simulink model "sdf_pi_test"  (R2018b)
settings: Solver=FixedStepAuto  StartTime=0.0  StopTime=60  FixedStep=tSample  RelTol=1e-3
PreLoadFcn:
  | init
values from neighbouring files (symbols this model uses):
  tSample = 1/fSample    (= 0.1)    [Ekf.m]    (also in init.m)
undefined symbols (not defined in the file or in its folder): X, Y, Z
libraries: robotlib x2
settings Model: Creator=HannesDittmann  LastModifiedBy=HannesDittmann

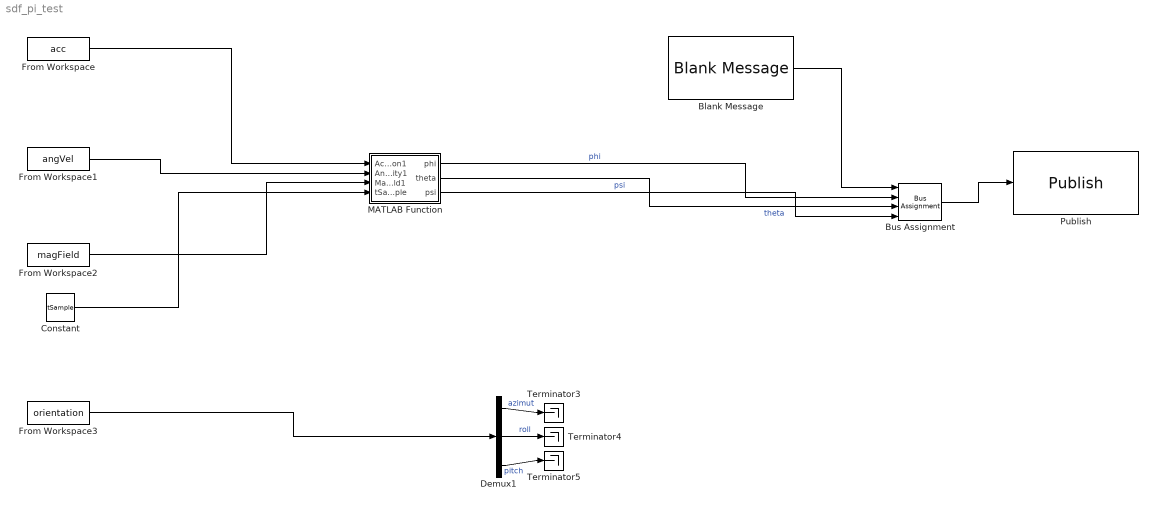
== system sdf_pi_test ==
  Blank Message : robotlib/Blank Message  messageClass=Message  entityType=geometry_msgs/Point  messageType=geometry_msgs/Point  SampleTime=inf
      settings: SourceProductBaseCode=RO
  Bus Assignment : BusAssignment  AssignedSignals=X,Y,Z
  Constant : Constant  Value=tSample
  Demux1 : Demux  Outputs=3
  From Workspace : FromWorkspace  VariableName=acc  Interpolate=off  OutputAfterFinalValue=Setting to zero
  From Workspace1 : FromWorkspace  VariableName=angVel  Interpolate=off  OutputAfterFinalValue=Setting to zero
  From Workspace2 : FromWorkspace  VariableName=magField  Interpolate=off  OutputAfterFinalValue=Setting to zero
  From Workspace3 : FromWorkspace  VariableName=orientation  Interpolate=off  OutputAfterFinalValue=Setting to zero
  MATLAB Function : MATLAB Function  TreatAsAtomicUnit=on
  Publish : robotlib/Publish  topicSource=Specify your own  topic=/euler  messageType=geometry_msgs/Point  messageQueueLength=1
      settings: SourceProductBaseCode=RO
  Terminator3 : Terminator
  Terminator4 : Terminator
  Terminator5 : Terminator
  wires:
  From Workspace/1 -> MATLAB Function/1(Acceleration1)
  From Workspace1/1 -> MATLAB Function/2(AngularVelocity1)
  From Workspace2/1 -> MATLAB Function/3(MagneticField1)
  Constant/1 -> MATLAB Function/4(tSample)
  From Workspace3/1 -> Demux1/1
  MATLAB Function/1(phi) -> Bus Assignment/2  "phi"
  MATLAB Function/2(theta) -> Bus Assignment/3  "theta"
  MATLAB Function/3(psi) -> Bus Assignment/4  "psi"
  Demux1/1 -> Terminator3/1  "azimut"
  Demux1/2 -> Terminator4/1  "roll"
  Demux1/3 -> Terminator5/1  "pitch"
  Blank Message/1 -> Bus Assignment/1
  Bus Assignment/1 -> Publish/1

== matlab function sdf_pi_test/MATLAB Function ==
  data: Acceleration1 input; phi output; AngularVelocity1 input; MagneticField1 input; tSample input; theta output; psi output
function [phi,theta,psi] = fcn(Acceleration1,AngularVelocity1,MagneticField1,tSample)


persistent x_dach P Q R C I

persistent firstRun

if isempty(firstRun)
  firstRun = 1;
  
    I=eye(3);

    C=I;

    P = 100*I;

R=[0.1 0 0;
   0 0.1 0;
   0 0 100];

Q=[.01 0 0;
   0 .0001 0;
   0 0 0.001];

x_dach = [0 0 0]'; % Startwerte phi theta psi

end


A_d = Ajacob(x_dach,AngularVelocity1,tSample,I);

[phi,theta,psi] = EulerAccel(Acceleration1(1),Acceleration1(2),MagneticField1);

[xp1 xp2 xp3] = fx(x_dach,AngularVelocity1,tSample);

Pp = A_d*P*A_d' + Q;    

K = Pp*C'*inv(C*Pp*C' + R);

x_dach = [xp1 xp2 xp3]' + K*([phi theta psi]' - C*[xp1 xp2 xp3]');
P = Pp - K*C*Pp;
 
phi=x_dach(1)*180/pi;
theta=x_dach(2)*180/pi;
psi=-x_dach(3)*180/pi;

end

function [phi,theta,psi] = EulerAccel(ax, ay, magnet)
%
%
g = 9.81; % Erdbeschleunigung in m/(s^2)


% Rückgabewerte sind die Eulerwinkel
theta = asin(  ax / g  );
phi   = asin( -ay /(g*cos(theta)));

xm=magnet(1);
ym=magnet(2);
zm=magnet(3);

xh = xm*cos(theta)+zm*sin(theta);
yh = xm*sin(phi)*sin(theta)+ym*cos(phi)-zm*sin(phi)*cos(theta);


psi = atan(yh/xh);

end



function [xp1 xp2 xp3] = fx(xhat, rates, dt)
%
%
phi   = xhat(1);
theta = xhat(2);

p = rates(1);
q = rates(2);
r = rates(3);

xdot = zeros(3, 1);

xdot(1) = p + q*sin(phi)*tan(theta) + r*cos(phi)*tan(theta);
xdot(2) =     q*cos(phi)            - r*sin(phi);
xdot(3) =     q*sin(phi)/cos(theta) + r*cos(phi)/cos(theta);

xp1 = xhat(1) + xdot(1)*dt; % Prädiktion des Zustandsvektors
xp2 = xhat(2) + xdot(2)*dt;
xp3 = xhat(3) + xdot(3)*dt;

end
